simulink model "proiectv5"  (Simulink 7.4)
settings: Solver=ode23tb  StartTime=0.0  StopTime=0.1  MaxStep=100e-6  RelTol=1e-3
libraries: powerlib x11
settings Model: Creator=Cristi  LastModifiedBy=Cristi

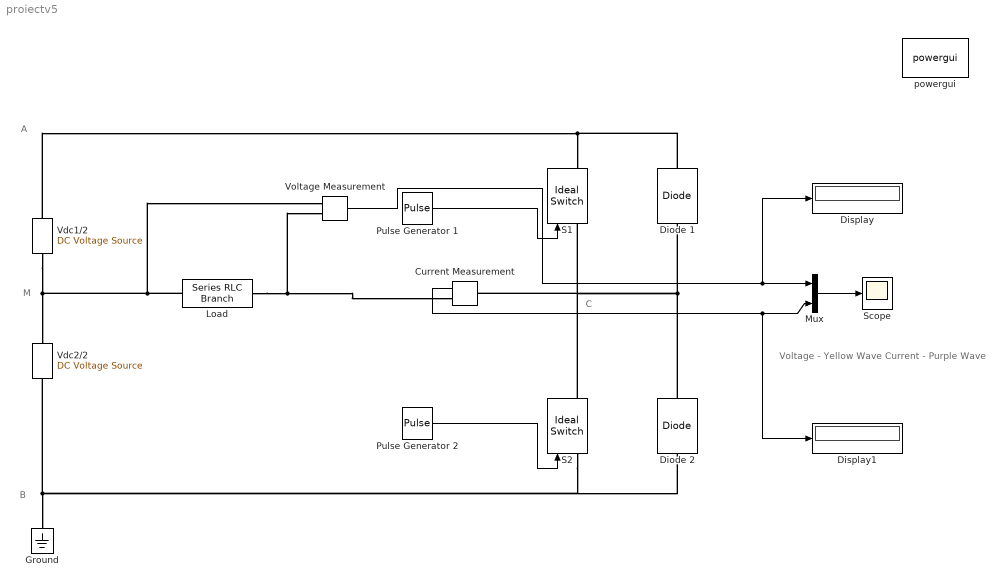
== system proiectv5 ==
  note: Voltage - Yellow Wave
      | Current - Purple Wave
  note: A
  note: B
  note: M
  note: C
  Current Measurement : powerlib/Measurements/Current Measurement  DialogController=POWERSYS.PowerSysDialog  SystemSampleTime=-1  PhasorSimulation=off  OutputType=Complex  PSBequivalent=0
  Diode 1 : powerlib/Power Electronics/Diode  DialogController=POWERSYS.PowerSysDialog  SystemSampleTime=-1  Ron=0.001  Lon=0  Vf=0.7  IC=0  UseSnubber=off  Rs=500  Cs=250e-9  Measurements=off
  Diode 2 : powerlib/Power Electronics/Diode  DialogController=POWERSYS.PowerSysDialog  SystemSampleTime=-1  Ron=0.001  Lon=0  Vf=0.7  IC=0  UseSnubber=off  Rs=500  Cs=250e-9  Measurements=off
  Display : Display
  Display1 : Display
  Ground : powerlib/Elements/Ground  DialogController=POWERSYS.PowerSysDialog  PhysicalDomain=powersysdomain  SubClassName=unknown  LeftPortType=p1  RightPortType=p1  LConnTagsString=a
  Load : powerlib/Elements/Series RLC Branch  DialogController=POWERSYS.PowerSysDialog  PhysicalDomain=powersysdomain  SubClassName=unknown  LeftPortType=p1  RightPortType=p1  LConnTagsString=__new0  RConnTagsString=__new0  BranchType=R  Resistance=1.5  Inductance=1e-3  SetiL0=off  InitialCurrent=0  Capacitance=1e-6  Setx0=off  InitialVoltage=0  Measurements=None
  Mux : Mux  Inputs=2
  Pulse Generator 1 : DiscretePulseGenerator  PulseType=Time based  Amplitude=115  Period=0.02  PulseWidth=50  PhaseDelay=0.01  SampleTime=1
  Pulse Generator 2 : DiscretePulseGenerator  PulseType=Time based  Amplitude=115  Period=0.02  PulseWidth=50  PhaseDelay=0  SampleTime=1
  S1 : powerlib/Power Electronics/Ideal Switch  DialogController=POWERSYS.PowerSysDialog  SystemSampleTime=-1  Ron=0.001  Lon=0  IC=0  Rs=1e5  Cs=inf  Measurements=on
  S2 : powerlib/Power Electronics/Ideal Switch  DialogController=POWERSYS.PowerSysDialog  SystemSampleTime=-1  Ron=0.001  Lon=0  IC=1  Rs=1e5  Cs=inf  Measurements=on
  Scope : Scope
      settings: TimeRange=0.1  DataFormat=Array
  Vdc1/2 : powerlib/Electrical Sources/DC Voltage Source  DialogController=POWERSYS.PowerSysDialog  SystemSampleTime=-1  Amplitude=115  Measurements=None
  Vdc2/2 : powerlib/Electrical Sources/DC Voltage Source  DialogController=POWERSYS.PowerSysDialog  SystemSampleTime=-1  Amplitude=115  Measurements=None
  Voltage Measurement : powerlib/Measurements/Voltage Measurement  DialogController=POWERSYS.PowerSysDialog  SystemSampleTime=-1  PhasorSimulation=off  OutputType=Complex  PSBequivalent=0
  powergui : powerlib/powergui  Priority=1  SystemSampleTime=-1  SimulationMode=Continuous  SampleTime=50e-6  frequency=60  SPID=off  DisableSnubberDevices=off  DisableRonSwitches=off  DisableVfSwitches=off  SwTol=0  Interpol=off  frequencyindice=0  echomessages=off  HookPort=off  DisplayEquations=off  FunctionMessages=off  EnableUseOfTLC=off  x0status=blocks  RestoreLinks=warning  Frange=[0:2:500]  Ylog=off  Xlog=on  ShowGrid=off  save=off  variable=ZData  structure=ScopeData  ZoomFFT=off  StartTime=0.0  cycles=1  DisplayStyle=3  fundamental=50  FreqAxis=off  MaxFrequency=1000  frequencyindicesteady=1  RmsSteady=1  display=off  Ts=0  methode=off
  wires:
  Pulse Generator 1/1 -> S1/1
  Pulse Generator 2/1 -> S2/1
  Mux/1 -> Scope/1
  Current Measurement/1 -> Mux/2, Display1/1
  Voltage Measurement/1 -> Mux/1, Display/1
  connections:
  S2/LConn1 -- Diode 2/LConn1 -- Vdc2/2/LConn1 -- Ground/LConn1
  Diode 1/RConn1 -- S1/RConn1 -- Vdc1/2/RConn1
  Load/LConn1 -- Vdc1/2/LConn1 -- Vdc2/2/RConn1 -- Voltage Measurement/LConn1
  Diode 2/RConn1 -- S1/LConn1 -- S2/RConn1 -- Current Measurement/LConn1 -- Diode 1/LConn1
  Load/RConn1 -- Current Measurement/RConn1 -- Voltage Measurement/LConn2
